simulink model "DC_DC_source_based_matrix_switches1"  (R2023b)
settings: Solver=FixedStepAuto  StartTime=0.0  StopTime=10000  FixedStep=0.01  RelTol=1e-3
InitFcn:
  | %run('D:\Thesis\main.m')
  | %run('E:\Thesis\main.m')
values from neighbouring files (symbols this model uses):
  cell_cap_Ah = 2.2    [find_maximum_ovlp.m]    (also in main.m)
  dst_q_cls = zeros(50, 2)    [main.m]
  dst_trg_soc_av = zeros(50, 1)    [main.m]
  soc = soc_in    [balance_costF.m]    (also in find_maximum_ovlp.m = fix(rand (1, cell_count) * 100); log_clustering.m; main.m = [16   16  50  27  27  23  22  73  73]; plot_final.m)
  src_q_cls = zeros(50, 2)    [main.m]
  src_trg_soc_av = zeros(50, 1)    [main.m]
undefined symbols (not defined in the file or in its folder): Ion, Lithium
libraries: spsIdealSwitchLib x18, spsBatteryLib x10, spsControlledCurrentSourceLib x4, spsVoltageMeasurementLib x4, simulink x2, slpidlib x1, spspowerguiLib x1
(part 1 of 2)
settings Model: NumberOfSteps=500  Creator=Mahdi  LastModifiedBy=Mahdi
settings OptimizationCC: DefaultParameterBehavior=Inlined  EnhancedBackFolding=on  PassReuseOutputArgsAs=Individual arguments  ZeroExternalMemoryAtStartup=off  ZeroInternalMemoryAtStartup=off  OptimizeBlockOrder=speed  DifferentSizesBufferReuse=on  OptimizationCustomize=off  EfficientTunableParamExpr=on
settings DebuggingCC: ParameterTunabilityLossMsg=error
settings HardwareCC: ProdBitPerInt=16  ProdBitPerPointer=16  ProdBitPerSizeT=16  ProdBitPerPtrDiffT=16  ProdLargestAtomicFloat=None  ProdWordSize=16  ProdHWDeviceType=STMicroelectronics->ST10/Super10
settings ModelReferenceCC: ModelReferenceMinAlgLoopOccurrences=on
settings SFSimCC: MATLABDynamicMemAlloc=off
settings RTWCC: Description=Embedded Coder  SystemTargetFile=ert.tlc  TemplateMakefile=ert_default_tmf
settings CodeAppCC: ForceParamTrailComments=on  IgnoreCustomStorageClasses=off  OperatorAnnotations=on  SimulinkDataObjDesc=on  SFDataObjDesc=on  InsertBlockDesc=on
settings ERTTargetCC: TargetLangStandard=C99 (ISO)  GenerateSampleERTMain=on  SupportContinuousTime=on  SupportVariableSizeSignals=on  InlinedParameterPlacement=NonHierarchical  ERTCustomFileTemplate=example_file_process.tlc

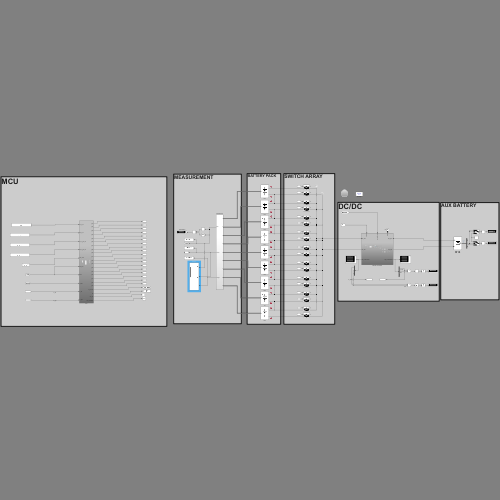
[thumbnail: Simulink's stored preview of the top-level diagram]
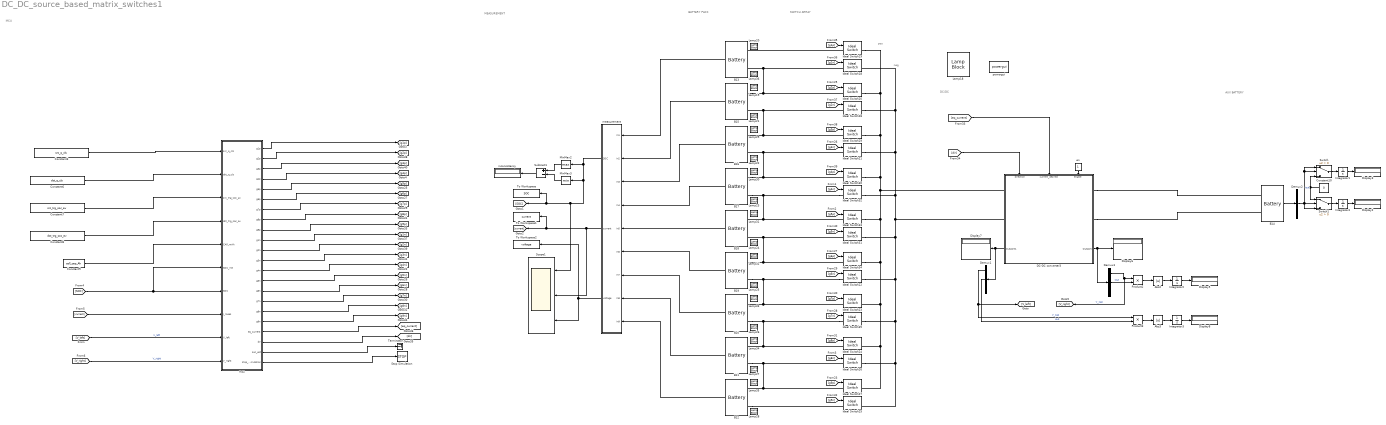
== system DC_DC_source_based_matrix_switches1 ==
  note: MEASUREMENT
  note: DC/DC
  note: SWITCH ARRAY
  note: pos
  note: BATTERY PACK
  note: neg
  note: AUX BATTERY
  note: MCU
  Abs2 : Abs  SaturateOnIntegerOverflow=off
  Abs3 : Abs  SaturateOnIntegerOverflow=off
  B11 : spsBatteryLib/Battery  BatType=Lithium-Ion  ShowTempParam=off  ThermalPreset=no  ShowAgeParam=off  NomV=3.7  NomQ=2.2  SOC=soc(1, 8)  Batt_Tr=30  PresetModel=on  MaxQ=2.2  MinV=2.775  FullV=4.3068  Dis_rate=0.95652  R=0.016818  Normal_OP=1.9896  expZone="[3.9974     0.10809]"  current=[6.5 13 32.5]  Units=Time  Tci=20  NomT=20  T2=-30  MaxQ2=4.8  FullV2=7.1  Normal_OP2=5.655  expZone2="[6.58           1]"  Rca=0.6  ti=2000  Dp=0  Neq0=0  Tsim=1e6  Ta1=25  Qeol=5.4*0.9  Reol=0.013333*1.2  Char_age=[2.3478, 3]  Dis_age=[2.3478, 10]  N1=1500  N2=10500  N3=1000  N4=1400  Ta2=45  N5=950
  B12 : spsBatteryLib/Battery  BatType=Lithium-Ion  ShowTempParam=off  ThermalPreset=no  ShowAgeParam=off  NomV=3.7  NomQ=2.2  SOC=soc(1, 9)  Batt_Tr=30  PresetModel=on  MaxQ=2.2  MinV=2.775  FullV=4.3068  Dis_rate=0.95652  R=0.016818  Normal_OP=1.9896  expZone="[3.9974     0.10809]"  current=[6.5 13 32.5]  Units=Time  Tci=20  NomT=20  T2=-30  MaxQ2=4.8  FullV2=7.1  Normal_OP2=5.655  expZone2="[6.58           1]"  Rca=0.6  ti=2000  Dp=0  Neq0=0  Tsim=1e6  Ta1=25  Qeol=5.4*0.9  Reol=0.013333*1.2  Char_age=[2.3478, 3]  Dis_age=[2.3478, 10]  N1=1500  N2=10500  N3=1000  N4=1400  Ta2=45  N5=950
  B13 : spsBatteryLib/Battery  BatType=Lithium-Ion  ShowTempParam=off  ThermalPreset=no  ShowAgeParam=off  NomV=3.7  NomQ=2.2  SOC=soc(1, 1)  Batt_Tr=30  PresetModel=on  MaxQ=2.2  MinV=2.775  FullV=4.3068  Dis_rate=0.95652  R=0.016818  Normal_OP=1.9896  expZone="[3.9974     0.10809]"  current=[6.5 13 32.5]  Units=Time  Tci=20  NomT=20  T2=-30  MaxQ2=4.8  FullV2=7.1  Normal_OP2=5.655  expZone2="[6.58           1]"  Rca=0.6  ti=2000  Dp=0  Neq0=0  Tsim=1e6  Ta1=25  Qeol=5.4*0.9  Reol=0.013333*1.2  Char_age=[2.3478, 3]  Dis_age=[2.3478, 10]  N1=1500  N2=10500  N3=1000  N4=1400  Ta2=45  N5=950
  B14 : spsBatteryLib/Battery  BatType=Lithium-Ion  ShowTempParam=off  ThermalPreset=no  ShowAgeParam=off  NomV=12  NomQ=60  SOC=soc(1, 1)  Batt_Tr=30  PresetModel=on  MaxQ=60  MinV=9  FullV=13.9678  Dis_rate=26.087  R=0.002  Normal_OP=54.2609  expZone="[12.9646      2.94783]"  current=[6.5 13 32.5]  Units=Time  Tci=20  NomT=20  T2=-30  MaxQ2=4.8  FullV2=7.1  Normal_OP2=5.655  expZone2="[6.58           1]"  Rca=0.6  ti=2000  Dp=0  Neq0=0  Tsim=1e6  Ta1=25  Qeol=5.4*0.9  Reol=0.013333*1.2  Char_age=[2.3478, 3]  Dis_age=[2.3478, 10]  N1=1500  N2=10500  N3=1000  N4=1400  Ta2=45  N5=950
  B15 : spsBatteryLib/Battery  BatType=Lithium-Ion  ShowTempParam=off  ThermalPreset=no  ShowAgeParam=off  NomV=3.7  NomQ=2.2  SOC=soc(1, 2)  Batt_Tr=30  PresetModel=on  MaxQ=2.2  MinV=2.775  FullV=4.3068  Dis_rate=0.95652  R=0.016818  Normal_OP=1.9896  expZone="[3.9974     0.10809]"  current=[6.5 13 32.5]  Units=Time  Tci=20  NomT=20  T2=-30  MaxQ2=4.8  FullV2=7.1  Normal_OP2=5.655  expZone2="[6.58           1]"  Rca=0.6  ti=2000  Dp=0  Neq0=0  Tsim=1e6  Ta1=25  Qeol=5.4*0.9  Reol=0.013333*1.2  Char_age=[2.3478, 3]  Dis_age=[2.3478, 10]  N1=1500  N2=10500  N3=1000  N4=1400  Ta2=45  N5=950
  B16 : spsBatteryLib/Battery  BatType=Lithium-Ion  ShowTempParam=off  ThermalPreset=no  ShowAgeParam=off  NomV=3.7  NomQ=2.2  SOC=soc(1, 3)  Batt_Tr=30  PresetModel=on  MaxQ=2.2  MinV=2.775  FullV=4.3068  Dis_rate=0.95652  R=0.016818  Normal_OP=1.9896  expZone="[3.9974     0.10809]"  current=[6.5 13 32.5]  Units=Time  Tci=20  NomT=20  T2=-30  MaxQ2=4.8  FullV2=7.1  Normal_OP2=5.655  expZone2="[6.58           1]"  Rca=0.6  ti=2000  Dp=0  Neq0=0  Tsim=1e6  Ta1=25  Qeol=5.4*0.9  Reol=0.013333*1.2  Char_age=[2.3478, 3]  Dis_age=[2.3478, 10]  N1=1500  N2=10500  N3=1000  N4=1400  Ta2=45  N5=950
  B17 : spsBatteryLib/Battery  BatType=Lithium-Ion  ShowTempParam=off  ThermalPreset=no  ShowAgeParam=off  NomV=3.7  NomQ=2.2  SOC=soc(1, 4)  Batt_Tr=30  PresetModel=on  MaxQ=2.2  MinV=2.775  FullV=4.3068  Dis_rate=0.95652  R=0.016818  Normal_OP=1.9896  expZone="[3.9974     0.10809]"  current=[6.5 13 32.5]  Units=Time  Tci=20  NomT=20  T2=-30  MaxQ2=4.8  FullV2=7.1  Normal_OP2=5.655  expZone2="[6.58           1]"  Rca=0.6  ti=2000  Dp=0  Neq0=0  Tsim=1e6  Ta1=25  Qeol=5.4*0.9  Reol=0.013333*1.2  Char_age=[2.3478, 3]  Dis_age=[2.3478, 10]  N1=1500  N2=10500  N3=1000  N4=1400  Ta2=45  N5=950
  B18 : spsBatteryLib/Battery  BatType=Lithium-Ion  ShowTempParam=off  ThermalPreset=no  ShowAgeParam=off  NomV=3.7  NomQ=2.2  SOC=soc(1, 5)  Batt_Tr=30  PresetModel=on  MaxQ=2.2  MinV=2.775  FullV=4.3068  Dis_rate=0.95652  R=0.016818  Normal_OP=1.9896  expZone="[3.9974     0.10809]"  current=[6.5 13 32.5]  Units=Time  Tci=20  NomT=20  T2=-30  MaxQ2=4.8  FullV2=7.1  Normal_OP2=5.655  expZone2="[6.58           1]"  Rca=0.6  ti=2000  Dp=0  Neq0=0  Tsim=1e6  Ta1=25  Qeol=5.4*0.9  Reol=0.013333*1.2  Char_age=[2.3478, 3]  Dis_age=[2.3478, 10]  N1=1500  N2=10500  N3=1000  N4=1400  Ta2=45  N5=950
  B19 : spsBatteryLib/Battery  BatType=Lithium-Ion  ShowTempParam=off  ThermalPreset=no  ShowAgeParam=off  NomV=3.7  NomQ=2.2  SOC=soc(1, 6)  Batt_Tr=30  PresetModel=on  MaxQ=2.2  MinV=2.775  FullV=4.3068  Dis_rate=0.95652  R=0.016818  Normal_OP=1.9896  expZone="[3.9974     0.10809]"  current=[6.5 13 32.5]  Units=Time  Tci=20  NomT=20  T2=-30  MaxQ2=4.8  FullV2=7.1  Normal_OP2=5.655  expZone2="[6.58           1]"  Rca=0.6  ti=2000  Dp=0  Neq0=0  Tsim=1e6  Ta1=25  Qeol=5.4*0.9  Reol=0.013333*1.2  Char_age=[2.3478, 3]  Dis_age=[2.3478, 10]  N1=1500  N2=10500  N3=1000  N4=1400  Ta2=45  N5=950
  B20 : spsBatteryLib/Battery  BatType=Lithium-Ion  ShowTempParam=off  ThermalPreset=no  ShowAgeParam=off  NomV=3.7  NomQ=2.2  SOC=soc(1, 7)  Batt_Tr=30  PresetModel=on  MaxQ=2.2  MinV=2.775  FullV=4.3068  Dis_rate=0.95652  R=0.016818  Normal_OP=1.9896  expZone="[3.9974     0.10809]"  current=[6.5 13 32.5]  Units=Time  Tci=20  NomT=20  T2=-30  MaxQ2=4.8  FullV2=7.1  Normal_OP2=5.655  expZone2="[6.58           1]"  Rca=0.6  ti=2000  Dp=0  Neq0=0  Tsim=1e6  Ta1=25  Qeol=5.4*0.9  Reol=0.013333*1.2  Char_age=[2.3478, 3]  Dis_age=[2.3478, 10]  N1=1500  N2=10500  N3=1000  N4=1400  Ta2=45  N5=950
  Constant10 : Constant  Value=0
  Constant3 : Constant  Value=src_q_cls
  Constant6 : Constant  Value=dst_q_cls
  Constant7 : Constant  Value=src_trg_soc_av
  Constant8 : Constant  Value=dst_trg_soc_av
  Constant9 : Constant  Value=cell_cap_Ah
  DC-DC converter3 : Subsystem
      settings: PortSchema="{\"entries\":[{\"content\":{\"sides\":[{\"content\":{\"connectorIds\":[\"LConn1\",\"LConn2\",\"Out2\"]},\"type\":\"ConnectorPlacement.EquallySpacedRectSide\",\"uuid\":\"b8e9ea21-fc6f-4abe-9815-7c96c8754cc1\"},{\"content\":{\"connectorIds\":[\"RConn1\",\"RConn2\",\"Out1\"],\"side\":\"RIGHT\"},\"type\":\"ConnectorPlacement.EquallySpacedRectSide\",\"uuid\":\"546bb611-6f28-45af-a15a-a960a3093258\"},{\"content\":{\"connectorIds\":[\"In1\",\"In2\",\"In3\"],\"side\":\"TOP\"},\"type\":\"ConnectorPlacement.EquallySpacedRectSide\",\"uuid\":\"f1a81754-76ae-41da-bcef-17d54c1fc977\"}]},\"type\":\"ConnectorPlacement.EquallySpacedConnector\",\"uuid\":\"f395fac5-4dd1-431a-bb8e-7682cfb9cc98\"}],\"packageUris\":[\"http://schema.mathworks.com/mf0/Connector/R2020b\"],\"version\":\"1.0\"}"
  Demux1 : Demux  Outputs=3
  Demux2 : Demux  Outputs=3
  Demux3 : Demux  Outputs=3
  Display{2..3,5..8} (6 alike) : Display
  Ideal Switch{18..35} (18 alike) : spsIdealSwitchLib/Ideal Switch  Ron=0.001  Lon=0  IC=0  Rs=1e5  Cs=inf  Measurements=on
  Integrator{1..4} (4 alike) : Integrator
  Lamp{18..36} (19 alike) : LampBlock  LabelPosition=Hide
  MinMax2 : MinMax  Function=max
  MinMax3 : MinMax
  Product2 : Product
  Product3 : Product
  Scope1 : Scope  NumInputPorts=3
  Stop Simulation : Stop
  Subtract1 : Sum  Inputs=+-
  Switch : Switch  Criteria=u2 > Threshold  SaturateOnIntegerOverflow=off  InputSameDT=off
  Switch1 : Switch  Criteria=u2 > Threshold  SaturateOnIntegerOverflow=off  InputSameDT=off
  Terminator : Terminator
  To Workspace : ToWorkspace  VariableName=SOC  SaveFormat=Timeseries  SampleTime=-1
      settings: Decimation=10
  To Workspace1 : ToWorkspace  VariableName=current  SaveFormat=Timeseries  SampleTime=-1
      settings: Decimation=10
  To Workspace2 : ToWorkspace  VariableName=voltage  SaveFormat=Timeseries  SampleTime=-1
      settings: Decimation=10
  en : Constant
  inconsistency : Display
  mcu : Subsystem
  measurement : Subsystem
  powergui : spspowerguiLib/powergui  Priority=1  SimulationMode=Discrete  SampleTime=1E-1  frequency=60  Iterations=50  frequencyindice=0  Pbase=100e6  ErrMax=1e-4  UnitsV=kV  UnitsW=MW  buscounter=0  FunctionMessages=off  echomessages=off  EnableUseOfTLC=off  CurrentSourceSwitches=off  DisableSnubberDevices=off  DisableRonSwitches=off  DisableVfSwitches=off  DisplayEquations=off  AutomaticDiscreteSolvers=off  SolverType=Tustin/Backward Euler (TBE)  Interpol=off  ExternalGateDelay=off  methode=on  Ts=1000  x0status=blocks  SPID=off  SwTol=0  HookPort=off  NonlinearTolerance=1e-4  nMaxIteration=10  ContinueOnMaxIteration=off  RestoreLinks=warning  ResistiveCurrentMeasurement=off  Frange=[0:2:500]  Ylog=off  Xlog=on  ShowGrid=off  save=off  variable=ZData  structure=0  ZoomFFT=off  StartTime=0.0  cycles=1  DisplayStyle=1  fundamental=60  FreqAxis=off  MaxFrequency=1000  frequencyindicesteady=1  RmsSteady=1  display=off
  wires:
  [g8n] -> Ideal Switch26/1
  Demux3/2 -> Product2/2  "Iout"
  measurement/1(SOC) -> MinMax2/1, MinMax3/1, Scope1/1, To Workspace/1, [SOC]
  [g2n] -> Ideal Switch28/1
  B11/1 -> measurement/8(In8)
  [g6n] -> Ideal Switch22/1
  MinMax3/1 -> Subtract1/2
  Demux1/2 -> Product3/2  "Iout"
  Product3/1 -> Abs3/1
  Subtract1/1 -> inconsistency/1
  [g9p] -> Ideal Switch27/1
  [g6p] -> Ideal Switch34/1
  B12/1 -> measurement/9(In9)
  [g5n] -> Ideal Switch31/1
  B20/1 -> measurement/7(In7)
  Demux1/1 -> [V_left], Product3/1  "V_cap"
  B19/1 -> measurement/6(In6)
  [g2p] -> Ideal Switch20/1
  [g8p] -> Ideal Switch24/1
  Abs2/1 -> Integrator2/1
  B15/1 -> measurement/2(In2)
  [g7n] -> Ideal Switch35/1
  [g4n] -> Ideal Switch32/1
  [g4p] -> Ideal Switch30/1
  measurement/2(current) -> Scope1/2, To Workspace1/1, [current]
  B18/1 -> measurement/5(In5)
  Product2/1 -> Abs2/1
  DC-DC converter3/1(Outport) -> Display6/1, Demux3/1
  MinMax2/1 -> Subtract1/1
  Integrator2/1 -> Display5/1
  [g1n] -> Ideal Switch18/1
  Integrator3/1 -> Display8/1
  Abs3/1 -> Integrator3/1
  [g5p] -> Ideal Switch33/1
  [g9n] -> Ideal Switch25/1
  B16/1 -> measurement/3(In3)
  [g1p] -> Ideal Switch19/1
  B17/1 -> measurement/4(In4)
  B13/1 -> measurement/1(In1)
  DC-DC converter3/2(Outport1) -> Display7/1, Demux1/1
  Demux3/1 -> [V_right], Product2/1  "V_cap"
  [g3p] -> Ideal Switch29/1
  [g3n] -> Ideal Switch21/1
  [g7p] -> Ideal Switch23/1
  measurement/3(voltage) -> To Workspace2/1, Scope1/3
  Integrator1/1 -> Display3/1
  Switch/1 -> Integrator1/1
  Integrator4/1 -> Display2/1
  B14/1 -> Demux2/1
  Demux2/2 -> Switch1/3, Switch1/2, Switch/1, Switch/2  "Iout"
  Switch1/1 -> Integrator4/1
  Constant10/1 -> Switch1/1, Switch/3
  [dir] -> DC-DC converter3/1(direction)
  en/1 -> DC-DC converter3/3(enable)
  Constant9/1 -> mcu/5(CAP_mAh)
  Constant7/1 -> mcu/3(src_trg_soc_av)
  Constant3/1 -> mcu/1(src_q_cls)
  Constant6/1 -> mcu/2(dst_q_cls)
  Constant8/1 -> mcu/4(dst_trg_soc_av)
  [SOC] -> mcu/6(SOC_init), mcu/7(SOC)
  [current] -> mcu/8(I_meas)
  mcu/13(g4n) -> [g4n]
  mcu/18(g9n) -> [g9n]
  mcu/19(eq_current) -> [eq_current]
  mcu/20(dir) -> [dir]
  mcu/17(g8n) -> [g8n]
  mcu/16(g7n) -> [g7n]
  mcu/15(g6n) -> [g6n]
  mcu/12(g3n) -> [g3n]
  mcu/14(g5n) -> [g5n]
  mcu/10(g1n) -> [g1n]
  mcu/11(g2n) -> [g2n]
  mcu/9(g9p) -> [g9p]
  mcu/8(g8p) -> [g8p]
  mcu/7(g7p) -> [g7p]
  mcu/6(g6p) -> [g6p]
  mcu/5(g5p) -> [g5p]
  mcu/4(g4p) -> [g4p]
  mcu/3(g3p) -> [g3p]
  mcu/2(g2p) -> [g2p]
  mcu/1(g1p) -> [g1p]
  mcu/21(soc_est) -> Terminator/1
  mcu/22(stop_simulation) -> Stop Simulation/1
  [eq_current] -> DC-DC converter3/2(current_desired)
  [V_left] -> mcu/9(V_left)  "V_left"
  [V_right] -> mcu/10(V_right)  "V_right"
  connections:
  B18/LConn2 -- Ideal Switch34/LConn1 -- B19/LConn1 -- Ideal Switch31/LConn1
  Ideal Switch29/RConn1 -- DC-DC converter3/LConn1 -- Ideal Switch23/RConn1 -- Ideal Switch27/RConn1 -- Ideal Switch24/RConn1 -- Ideal Switch34/RConn1 -- Ideal Switch33/RConn1 -- Ideal Switch30/RConn1 -- Ideal Switch19/RConn1 -- Ideal Switch20/RConn1
  Ideal Switch32/RConn1 -- Ideal Switch18/RConn1 -- Ideal Switch28/RConn1 -- Ideal Switch21/RConn1 -- DC-DC converter3/LConn2 -- Ideal Switch22/RConn1 -- Ideal Switch26/RConn1 -- Ideal Switch25/RConn1 -- Ideal Switch35/RConn1 -- Ideal Switch31/RConn1
  B15/LConn1 -- B13/LConn2 -- Ideal Switch18/LConn1 -- Ideal Switch20/LConn1
  Ideal Switch35/LConn1 -- Ideal Switch24/LConn1 -- B11/LConn1 -- B20/LConn2
  Ideal Switch21/LConn1 -- B16/LConn2 -- B17/LConn1 -- Ideal Switch30/LConn1
  Ideal Switch22/LConn1 -- B20/LConn1 -- Ideal Switch23/LConn1 -- B19/LConn2
  Ideal Switch32/LConn1 -- B18/LConn1 -- Ideal Switch33/LConn1 -- B17/LConn2
  Ideal Switch29/LConn1 -- B16/LConn1 -- Ideal Switch28/LConn1 -- B15/LConn2
  B12/LConn1 -- Ideal Switch27/LConn1 -- Ideal Switch26/LConn1 -- B11/LConn2
  Ideal Switch19/LConn1 -- B13/LConn1
  DC-DC converter3/RConn1 -- B14/LConn1
  B12/LConn2 -- Ideal Switch25/LConn1
  DC-DC converter3/RConn2 -- B14/LConn2

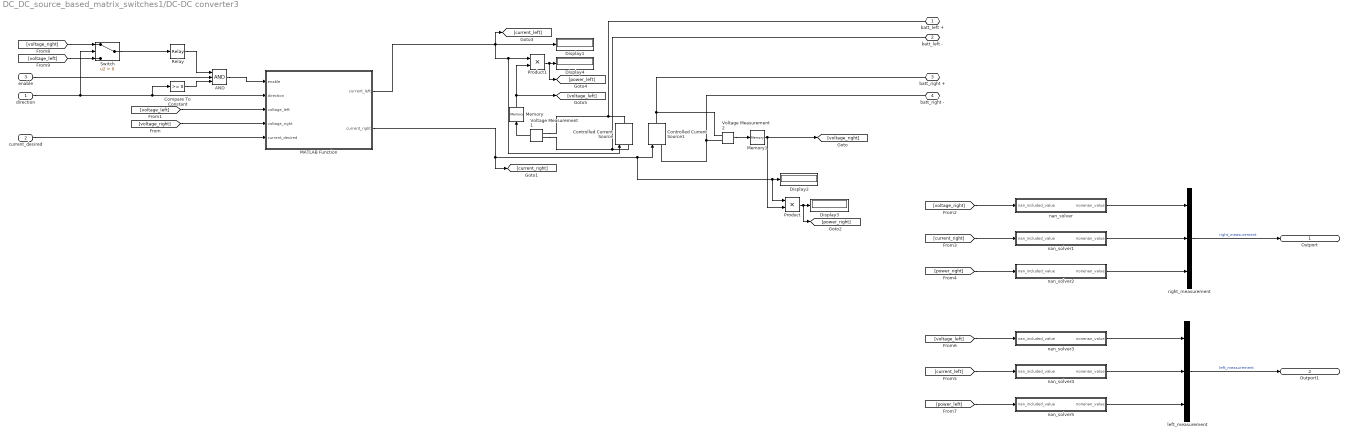
== system DC_DC_source_based_matrix_switches1/DC-DC converter3 ==
  direction : Inport
  current_desired : Inport  Port=2
  enable : Inport  Port=3
  AND : Logic  Inputs=3  IconShape=distinctive  AllPortsSameDT=off  OutDataTypeStr=boolean
  Compare To Constant : simulink/Logic and Bit Operations/Compare To Constant  relop=>=  const=0  OutDataTypeStr=boolean
  Controlled Current Source : spsControlledCurrentSourceLib/Controlled Current Source  Initialize=on  Source_Type=DC  Amplitude=0  Phase=0  Frequency=0  Measurements=None
  Controlled Current Source1 : spsControlledCurrentSourceLib/Controlled Current Source  Initialize=on  Source_Type=AC  Amplitude=0  Phase=0  Frequency=0  Measurements=None
  Display{1..4} (4 alike) : Display
  MATLAB Function : MATLAB Function  TreatAsAtomicUnit=on
  Memory : Memory
  Memory1 : Memory
  Product : Product
  Product1 : Product
  Relay : Relay  OnSwitchValue=3.5  OffSwitchValue=2
  Switch : Switch  Criteria=u2 > Threshold  SaturateOnIntegerOverflow=off  InputSameDT=off
  Voltage Measurement1 : spsVoltageMeasurementLib/Voltage Measurement  PhasorSimulation=off  OutputType=Complex  PSBequivalent=0
  Voltage Measurement2 : spsVoltageMeasurementLib/Voltage Measurement  PhasorSimulation=off  OutputType=Complex  PSBequivalent=0
  left_measurement : Mux  Inputs=3
  nan_solver : Subsystem
  nan_solver1 : Subsystem
  nan_solver2 : Subsystem
  nan_solver3 : Subsystem
  nan_solver4 : Subsystem
  nan_solver5 : Subsystem
  right_measurement : Mux  Inputs=3
  batt_left + : PMIOPort  Side=Left
  batt_left - : PMIOPort  Port=2  Side=Left
  batt_right + : PMIOPort  Port=3  Side=Right
  batt_right - : PMIOPort  Port=4  Side=Right
  Outport : Outport
  Outport1 : Outport  Port=2
  wires:
  MATLAB Function/1(current_left) -> Controlled Current Source/1, Product1/1, [current_left], Display1/1
  enable/1 -> AND/2
  Voltage Measurement2/1 -> Memory1/1
  direction/1 -> Compare To Constant/1, MATLAB Function/2(direction), Switch/2
  [voltage_right] -> MATLAB Function/4(voltage_right)
  [voltage_left] -> MATLAB Function/3(voltage_left)
  Product/1 -> [power_right], Display3/1
  Product1/1 -> [power_left], Display4/1
  [voltage_right] -> nan_solver/1(nan_included_value)
  [current_right] -> nan_solver1/1(nan_included_value)
  [power_right] -> nan_solver2/1(nan_included_value)
  [power_left] -> nan_solver5/1(nan_included_value)
  [current_left] -> nan_solver4/1(nan_included_value)
  [voltage_left] -> nan_solver3/1(nan_included_value)
  right_measurement/1 -> Outport/1  "right_measurement"
  left_measurement/1 -> Outport1/1  "left_measurement"
  Voltage Measurement1/1 -> Memory/1
  Relay/1 -> AND/1
  AND/1 -> MATLAB Function/1(enable)
  Switch/1 -> Relay/1
  [voltage_left] -> Switch/3
  [voltage_right] -> Switch/1
  Memory/1 -> Product1/2, [voltage_left]
  Memory1/1 -> [voltage_right], Product/2
  Compare To Constant/1 -> AND/3
  MATLAB Function/2(current_right) -> [current_right], Product/1, Display2/1, Controlled Current Source1/1
  current_desired/1 -> MATLAB Function/5(current_desired)
  nan_solver/1(nonenan_value) -> right_measurement/1
  nan_solver1/1(nonenan_value) -> right_measurement/2
  nan_solver2/1(nonenan_value) -> right_measurement/3
  nan_solver3/1(nonenan_value) -> left_measurement/1
  nan_solver4/1(nonenan_value) -> left_measurement/2
  nan_solver5/1(nonenan_value) -> left_measurement/3
  connections:
  Voltage Measurement1/LConn1 -- batt_left +/RConn1 -- Controlled Current Source/RConn1
  Controlled Current Source1/RConn1 -- batt_right +/RConn1 -- Voltage Measurement2/LConn1
  Voltage Measurement2/LConn2 -- Controlled Current Source1/LConn1 -- batt_right -/RConn1
  Voltage Measurement1/LConn2 -- batt_left -/RConn1 -- Controlled Current Source/LConn1

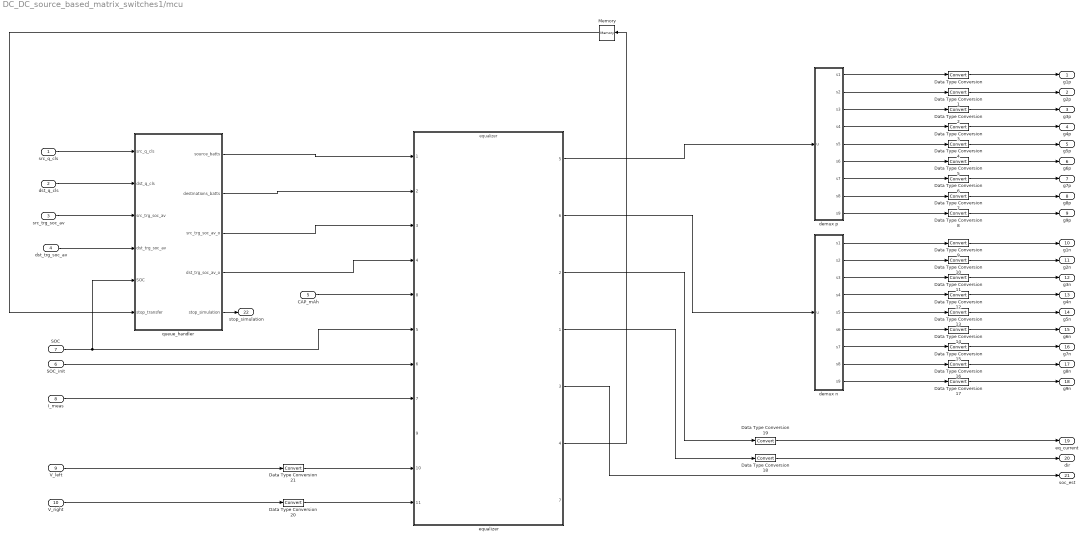
== system DC_DC_source_based_matrix_switches1/mcu ==
  src_q_cls : Inport
  dst_q_cls : Inport  Port=2
  src_trg_soc_av : Inport  Port=3
  dst_trg_soc_av : Inport  Port=4
  CAP_mAh : Inport  Port=5  PortDimensions=[1 1]
  SOC_init : Inport  Port=6
  SOC : Inport  Port=7
  I_meas : Inport  Port=8
  V_left : Inport  Port=9
  V_right : Inport  Port=10
  Data Type Conversion{,1..21} (22 alike) : DataTypeConversion  SaturateOnIntegerOverflow=off  RndMeth=Floor
  Memory : Memory
  demux n : MATLAB Function  TreatAsAtomicUnit=on
  demux p : MATLAB Function  TreatAsAtomicUnit=on
  equalizer : ModelReference  ModelNameDialog=equalizer.slx  SimulationMode=Normal  ModelReferenceVersion=4.57
      settings: PortSchema="{\"entries\":[{\"content\":{\"sides\":[{\"content\":{\"connectorIds\":[\"In1\",\"In2\",\"In3\",\"In4\",\"In8\",\"In5\",\"In6\",\"In7\",\"In9\",\"In10\",\"In11\"]},\"type\":\"ConnectorPlacement.EquallySpacedRectSide\",\"uuid\":\"0e6c575f-ddf8-42c7-9de1-4e19b4f5acff\"},{\"content\":{\"connectorIds\":[\"Out5\",\"Out6\",\"Out2\",\"Out1\",\"Out3\",\"Out4\",\"Out7\"],\"side\":\"RIGHT\"},\"type\":\"ConnectorPlacement.EquallySpacedRectSide\",\"uuid\":\"ffa8e601-c4c1-438b-9d74-db810c4522c7\"},{\"content\":{\"side\":\"TOP\"},\"type\":\"ConnectorPlacement.EquallySpacedRectSide\",\"uuid\":\"66088ef6-14ba-4cc7-bf73-23eeb83a4754\"}]},\"type\":\"ConnectorPlacement.EquallySpacedConnector\",\"uuid\":\"d6774570-3838-464e-8129-9c381a0fca30\"}],\"packageUris\":[\"http://schema.mathworks.com/mf0/Connector/R2020b\"],\"version\":\"1.0\"}"
  queue_handler : MATLAB Function  TreatAsAtomicUnit=on
  g1p : Outport  PortDimensions=1
  g2p : Outport  Port=2
  g3p : Outport  Port=3
  g4p : Outport  Port=4
  g5p : Outport  Port=5
  g6p : Outport  Port=6
  g7p : Outport  Port=7
  g8p : Outport  Port=8
  g9p : Outport  Port=9
  g1n : Outport  Port=10
  g2n : Outport  Port=11
  g3n : Outport  Port=12
  g4n : Outport  Port=13
  g5n : Outport  Port=14
  g6n : Outport  Port=15
  g7n : Outport  Port=16
  g8n : Outport  Port=17
  g9n : Outport  Port=18
  eq_current : Outport  Port=19
  dir : Outport  Port=20
  soc_est : Outport  Port=21  PortDimensions=[1 9]
  stop_simulation : Outport  Port=22  PortDimensions=1
  wires:
  equalizer/2 -> Data Type Conversion19/1
  equalizer/1 -> Data Type Conversion18/1
  equalizer/3 -> soc_est/1
  equalizer/4 -> Memory/1
  SOC/1 -> equalizer/5, queue_handler/5(SOC)
  SOC_init/1 -> equalizer/6
  I_meas/1 -> equalizer/7
  CAP_mAh/1 -> equalizer/8
  src_q_cls/1 -> queue_handler/1(src_q_cls)
  dst_q_cls/1 -> queue_handler/2(dst_q_cls)
  src_trg_soc_av/1 -> queue_handler/3(src_trg_soc_av)
  dst_trg_soc_av/1 -> queue_handler/4(dst_trg_soc_av)
  queue_handler/1(source_batts) -> equalizer/1
  queue_handler/2(destinations_batts) -> equalizer/2
  queue_handler/3(src_trg_soc_av_o) -> equalizer/3
  queue_handler/4(dst_trg_soc_av_o) -> equalizer/4
  Memory/1 -> queue_handler/6(stop_transfer)
  Data Type Conversion18/1 -> dir/1
  Data Type Conversion19/1 -> eq_current/1
  queue_handler/5(stop_simulation) -> stop_simulation/1
  Data Type Conversion/1 -> g1p/1
  Data Type Conversion1/1 -> g2p/1
  Data Type Conversion2/1 -> g3p/1
  Data Type Conversion3/1 -> g4p/1
  Data Type Conversion4/1 -> g5p/1
  Data Type Conversion5/1 -> g6p/1
  Data Type Conversion6/1 -> g7p/1
  Data Type Conversion7/1 -> g8p/1
  Data Type Conversion8/1 -> g9p/1
  Data Type Conversion9/1 -> g1n/1
  Data Type Conversion10/1 -> g2n/1
  Data Type Conversion11/1 -> g3n/1
  Data Type Conversion12/1 -> g4n/1
  Data Type Conversion13/1 -> g5n/1
  Data Type Conversion14/1 -> g6n/1
  Data Type Conversion15/1 -> g7n/1
  Data Type Conversion16/1 -> g8n/1
  Data Type Conversion17/1 -> g9n/1
  demux p/5(s5) -> Data Type Conversion4/1
  demux p/8(s8) -> Data Type Conversion7/1
  demux p/9(s9) -> Data Type Conversion8/1
  demux p/7(s7) -> Data Type Conversion6/1
  equalizer/6 -> demux n/1(u)
  demux p/4(s4) -> Data Type Conversion3/1
  demux p/1(s1) -> Data Type Conversion/1
  demux p/6(s6) -> Data Type Conversion5/1
  demux p/2(s2) -> Data Type Conversion1/1
  demux n/3(s3) -> Data Type Conversion11/1
  demux n/5(s5) -> Data Type Conversion13/1
  demux p/3(s3) -> Data Type Conversion2/1
  demux n/9(s9) -> Data Type Conversion17/1
  demux n/6(s6) -> Data Type Conversion14/1
  demux n/4(s4) -> Data Type Conversion12/1
  demux n/7(s7) -> Data Type Conversion15/1
  demux n/1(s1) -> Data Type Conversion9/1
  demux n/8(s8) -> Data Type Conversion16/1
  demux n/2(s2) -> Data Type Conversion10/1
  equalizer/5 -> demux p/1(u)
  V_left/1 -> Data Type Conversion21/1
  V_right/1 -> Data Type Conversion20/1
  Data Type Conversion21/1 -> equalizer/10
  Data Type Conversion20/1 -> equalizer/11

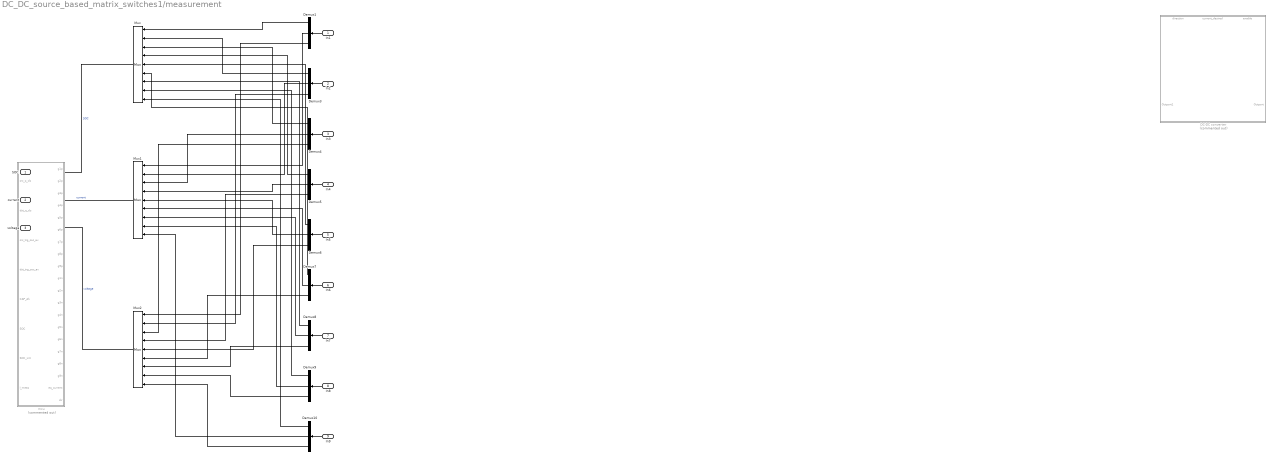
== system DC_DC_source_based_matrix_switches1/measurement ==
  In1 : Inport
  In2 : Inport  Port=2
  In3 : Inport  Port=3
  In4 : Inport  Port=4
  In5 : Inport  Port=5
  In6 : Inport  Port=6
  In7 : Inport  Port=7
  In8 : Inport  Port=8
  In9 : Inport  Port=9
  DC-DC converter : Subsystem  Commented=on
      settings: PortSchema="{\"entries\":[{\"content\":{\"sides\":[{\"content\":{\"connectorIds\":[\"LConn1\",\"LConn2\",\"Out2\"]},\"type\":\"ConnectorPlacement.EquallySpacedRectSide\",\"uuid\":\"b8e9ea21-fc6f-4abe-9815-7c96c8754cc1\"},{\"content\":{\"connectorIds\":[\"RConn1\",\"RConn2\",\"Out1\"],\"side\":\"RIGHT\"},\"type\":\"ConnectorPlacement.EquallySpacedRectSide\",\"uuid\":\"546bb611-6f28-45af-a15a-a960a3093258\"},{\"content\":{\"connectorIds\":[\"In1\",\"In2\",\"In3\"],\"side\":\"TOP\"},\"type\":\"ConnectorPlacement.EquallySpacedRectSide\",\"uuid\":\"f1a81754-76ae-41da-bcef-17d54c1fc977\"}]},\"type\":\"ConnectorPlacement.EquallySpacedConnector\",\"uuid\":\"f395fac5-4dd1-431a-bb8e-7682cfb9cc98\"}],\"packageUris\":[\"http://schema.mathworks.com/mf0/Connector/R2020b\"],\"version\":\"1.0\"}"
  Demux{1,3..10} (9 alike) : Demux  Outputs=3
  Mux : Mux  Inputs=9
  Mux1 : Mux  Inputs=9
  Mux2 : Mux  Inputs=9
  mcu : Subsystem  Commented=on
  SOC : Outport
  current : Outport  Port=2
  voltage : Outport  Port=3
  wires:
  In7/1 -> Demux8/1
  Demux6/3 -> Mux2/5
  Demux8/3 -> Mux2/7
  In5/1 -> Demux6/1
  Demux7/3 -> Mux2/6
  Demux4/1 -> Mux/3
  Demux10/3 -> Mux2/9
  Mux1/1 -> current/1  "current"
  Demux4/2 -> Mux1/3
  Demux1/3 -> Mux2/1
  Demux5/3 -> Mux2/4
  Demux10/1 -> Mux/9
  Demux4/3 -> Mux2/3
  Demux9/2 -> Mux1/8
  Demux9/3 -> Mux2/8
  Demux3/3 -> Mux2/2
  Demux9/1 -> Mux/8
  Demux10/2 -> Mux1/9
  Demux8/2 -> Mux1/7
  Demux3/1 -> Mux/2
  In6/1 -> Demux7/1
  Demux1/2 -> Mux1/1
  Demux6/1 -> Mux/5
  Demux8/1 -> Mux/7
  In1/1 -> Demux1/1
  In9/1 -> Demux10/1
  Demux7/1 -> Mux/6
  Demux1/1 -> Mux/1
  Demux3/2 -> Mux1/2
  Demux5/1 -> Mux/4
  Demux5/2 -> Mux1/4
  Demux6/2 -> Mux1/5
  Demux7/2 -> Mux1/6
  Mux/1 -> SOC/1  "SOC"
  In2/1 -> Demux3/1
  Mux2/1 -> voltage/1  "voltage"
  In3/1 -> Demux4/1
  In4/1 -> Demux5/1
  In8/1 -> Demux9/1

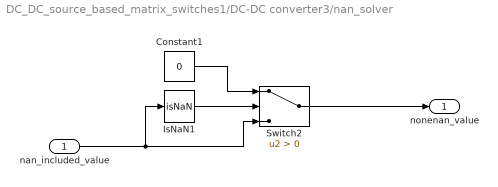
== system DC_DC_source_based_matrix_switches1/DC-DC converter3/nan_solver ==
  nan_included_value : Inport
  Constant1 : Constant  Value=0
  IsNaN1 : RelationalOperator  Operator=isNaN  OutDataTypeStr=boolean  RndMeth=Simplest  InputSameDT=off
  Switch2 : Switch  Criteria=u2 > Threshold  SaturateOnIntegerOverflow=off  InputSameDT=off
  nonenan_value : Outport
  wires:
  Constant1/1 -> Switch2/1
  nan_included_value/1 -> IsNaN1/1, Switch2/3
  IsNaN1/1 -> Switch2/2
  Switch2/1 -> nonenan_value/1

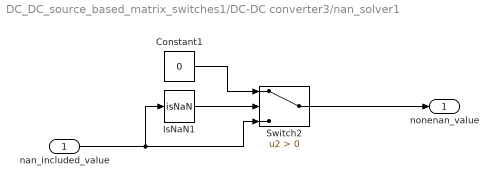
== system DC_DC_source_based_matrix_switches1/DC-DC converter3/nan_solver1 ==
  nan_included_value : Inport
  Constant1 : Constant  Value=0
  IsNaN1 : RelationalOperator  Operator=isNaN  OutDataTypeStr=boolean  RndMeth=Simplest  InputSameDT=off
  Switch2 : Switch  Criteria=u2 > Threshold  SaturateOnIntegerOverflow=off  InputSameDT=off
  nonenan_value : Outport
  wires:
  Switch2/1 -> nonenan_value/1
  IsNaN1/1 -> Switch2/2
  nan_included_value/1 -> Switch2/3, IsNaN1/1
  Constant1/1 -> Switch2/1

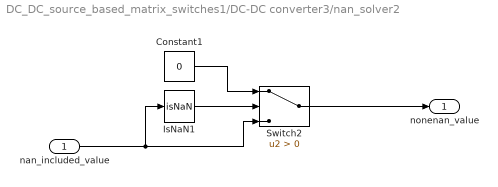
== system DC_DC_source_based_matrix_switches1/DC-DC converter3/nan_solver2 ==
  nan_included_value : Inport
  Constant1 : Constant  Value=0
  IsNaN1 : RelationalOperator  Operator=isNaN  OutDataTypeStr=boolean  RndMeth=Simplest  InputSameDT=off
  Switch2 : Switch  Criteria=u2 > Threshold  SaturateOnIntegerOverflow=off  InputSameDT=off
  nonenan_value : Outport
  wires:
  Constant1/1 -> Switch2/1
  nan_included_value/1 -> IsNaN1/1, Switch2/3
  IsNaN1/1 -> Switch2/2
  Switch2/1 -> nonenan_value/1

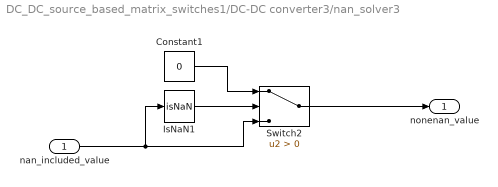
== system DC_DC_source_based_matrix_switches1/DC-DC converter3/nan_solver3 ==
  nan_included_value : Inport
  Constant1 : Constant  Value=0
  IsNaN1 : RelationalOperator  Operator=isNaN  OutDataTypeStr=boolean  RndMeth=Simplest  InputSameDT=off
  Switch2 : Switch  Criteria=u2 > Threshold  SaturateOnIntegerOverflow=off  InputSameDT=off
  nonenan_value : Outport
  wires:
  Switch2/1 -> nonenan_value/1
  IsNaN1/1 -> Switch2/2
  nan_included_value/1 -> Switch2/3, IsNaN1/1
  Constant1/1 -> Switch2/1

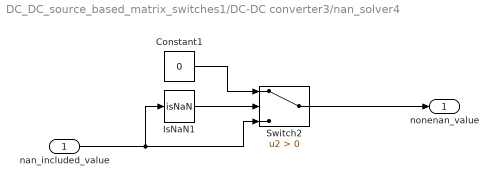
== system DC_DC_source_based_matrix_switches1/DC-DC converter3/nan_solver4 ==
  nan_included_value : Inport
  Constant1 : Constant  Value=0
  IsNaN1 : RelationalOperator  Operator=isNaN  OutDataTypeStr=boolean  RndMeth=Simplest  InputSameDT=off
  Switch2 : Switch  Criteria=u2 > Threshold  SaturateOnIntegerOverflow=off  InputSameDT=off
  nonenan_value : Outport
  wires:
  Constant1/1 -> Switch2/1
  nan_included_value/1 -> IsNaN1/1, Switch2/3
  IsNaN1/1 -> Switch2/2
  Switch2/1 -> nonenan_value/1

== system DC_DC_source_based_matrix_switches1/DC-DC converter3/nan_solver5 ==
  nan_included_value : Inport
  Constant1 : Constant  Value=0
  IsNaN1 : RelationalOperator  Operator=isNaN  OutDataTypeStr=boolean  RndMeth=Simplest  InputSameDT=off
  Switch2 : Switch  Criteria=u2 > Threshold  SaturateOnIntegerOverflow=off  InputSameDT=off
  nonenan_value : Outport
  wires:
  Switch2/1 -> nonenan_value/1
  IsNaN1/1 -> Switch2/2
  nan_included_value/1 -> Switch2/3, IsNaN1/1
  Constant1/1 -> Switch2/1

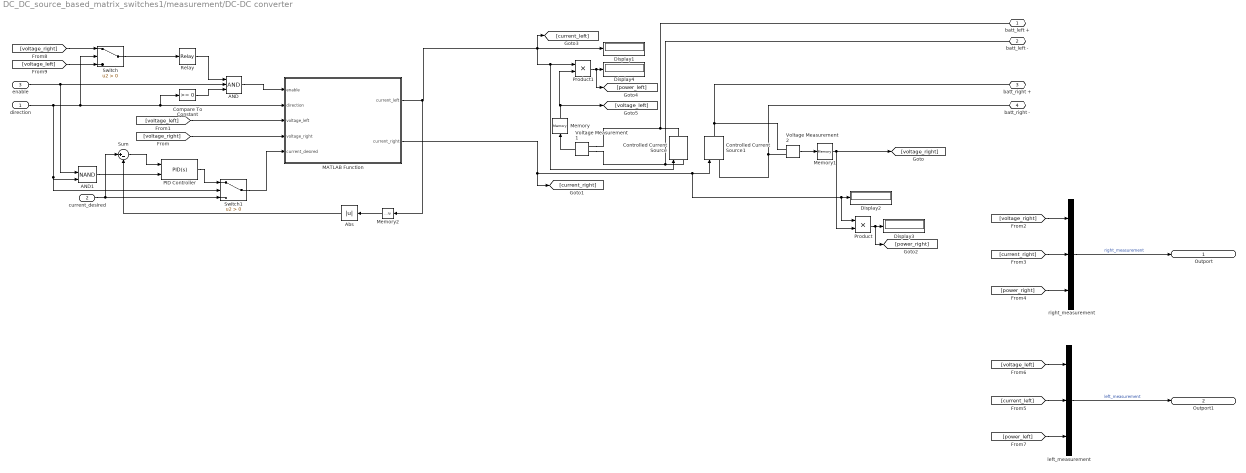
== system DC_DC_source_based_matrix_switches1/measurement/DC-DC converter ==
  direction : Inport
  current_desired : Inport  Port=2
  enable : Inport  Port=3
  AND : Logic  Inputs=3  IconShape=distinctive  AllPortsSameDT=off  OutDataTypeStr=boolean
  AND1 : Logic  Operator=NAND  IconShape=distinctive  AllPortsSameDT=off  OutDataTypeStr=boolean
  Abs : Abs  SaturateOnIntegerOverflow=off
  Compare To Constant : simulink/Logic and Bit Operations/Compare To Constant  relop=>=  const=0  OutDataTypeStr=boolean
  Controlled Current Source : spsControlledCurrentSourceLib/Controlled Current Source  Initialize=on  Source_Type=DC  Amplitude=0  Phase=0  Frequency=0  Measurements=None
  Controlled Current Source1 : spsControlledCurrentSourceLib/Controlled Current Source  Initialize=on  Source_Type=AC  Amplitude=0  Phase=0  Frequency=0  Measurements=None
  Display{1..4} (4 alike) : Display
  MATLAB Function : MATLAB Function  TreatAsAtomicUnit=on
  Memory : Memory
  Memory1 : Memory
  Memory2 : Memory
  PID Controller : slpidlib/PID Controller  Controller=PID  Form=Parallel  TimeDomain=Continuous-time  UseExternalTs=off  SampleTime=-1  IntegratorMethod=Forward Euler  FilterMethod=Forward Euler  ControllerParametersSource=internal  P=0.01  I=2  UseKiTs=off  D=0  N=100  UseFilter=on  TunerSelectOption=Transfer Function Based (PID Tuner App)  InitialConditionSource=internal  InitialConditionForIntegrator=0  InitialConditionForFilter=0  DifferentiatorICPrevScaledInput=0  ExternalReset=level  TrackingMode=off  Kt=1  LimitOutput=on  SatLimitsSource=internal  UpperSaturationLimit=2  LowerSaturationLimit=0  LinearizeAsGain=on  AntiWindupMode=none  Kb=1  LimitIntegrator=off  UpperIntegratorSaturationLimit=inf  LowerIntegratorSaturationLimit=-inf  POutMin=[]  POutMax=[]  IOutMin=[]  IOutMax=[]  DOutMin=[]  DOutMax=[]  NOutMin=[]  NOutMax=[]  SumOutMin=[]  SumOutMax=[]  SaturationOutMin=[]  SaturationOutMax=[]  PParamMin=[]  PParamMax=[]  IParamMin=[]  IParamMax=[]  DParamMin=[]  DParamMax=[]  NParamMin=[]  NParamMax=[]  KbParamMin=[]  KbParamMax=[]  KtParamMin=[]  KtParamMax=[]  KbOutMin=[]  KbOutMax=[]  KtOutMin=[]  KtOutMax=[]  IntegratorOutMin=[]  IntegratorOutMax=[]  FilterOutMin=[]  FilterOutMax=[]  SumI1OutMin=[]  SumI1OutMax=[]  SumI2OutMin=[]  SumI2OutMax=[]  SumI3OutMin=[]  SumI3OutMax=[]  SumI4OutMin=[]  SumI4OutMax=[]  SumDOutMin=[]  SumDOutMax=[]  DifferentiatorOutMin=[]  DifferentiatorOutMax=[]  FilterDiffOutCoefMin=[]  FilterDiffOutCoefMax=[]  ReciprocalOutMin=[]  ReciprocalOutMax=[]  SumDenOutMin=[]  SumDenOutMax=[]  SumNumOutMin=[]  SumNumOutMax=[]  DivideOutMin=[]  DivideOutMax=[]  UdiffTsProdOutMin=[]  UdiffTsProdOutMax=[]  NTsProdOutMin=[]  NTsProdOutMax=[]  UintegralTsProdOutMin=[]  UintegralTsProdOutMax=[]  UngainTsProdOutMin=[]  UngainTsProdOutMax=[]  ClampingZeroOutDataTypeStr=Inherit: Inherit via back propagation  ClampingZeroOutMin=[]  ClampingZeroOutMax=[]  FilterDenConstantOutDataTypeStr=Inherit: Inherit via back propagation  FilterDenConstantOutMin=[]  FilterDenConstantOutMax=[]  PCopyOutDataTypeStr=Inherit: Inherit via back propagation  PCopyOutMin=[]  PCopyOutMax=[]  NCopyOutDataTypeStr=Inherit: Inherit via back propagation  NCopyOutMin=[]  NCopyOutMax=[]  IntegratorContinuousStateAttributes=''  IntegratorStateMustResolveToSignalObject=off  IntegratorRTWStateStorageClass=Auto  FilterContinuousStateAttributes=''  FilterStateMustResolveToSignalObject=off  FilterRTWStateStorageClass=Auto  ParallelPVariant=InternalParameters  IdealPVariant=Disabled  IVariant=InternalParameters  DVariant=InternalParameters  IntegratorVariant=Continuous  SatVariant=Enabled  AWVariant=Passthrough  PCopyVariant=Disabled  TRVariant=Disabled  FdbkBlocksVariant=Forward  IdealPFdbkVariant=Disabled  SatFdbkVariant=Disabled  DerivativeFilterVariant=ContFilter  NVariant=InternalParameters  NCopyVariant=Disabled  FilterICVariant=InternalICsFilter  IntegratorICVariant=InternalICs  ExternalResetVariant=ExternalReset  TRSumVariant=Passthrough  SumFdbkVariant=Disabled  SumVariant=Sum_PID  TsampFilterVariant=InternalTs  TsampNgainVariant=Passthrough  TsampIntegralVariant=Disabled_SignalSpec  ExternalSaturationOutDataTypeStr=Inherit: Same as second input
  Product : Product
  Product1 : Product
  Relay : Relay  OnSwitchValue=3.5  OffSwitchValue=2
  Sum : Sum  Inputs=|+-
  Switch : Switch  Criteria=u2 > Threshold  SaturateOnIntegerOverflow=off  InputSameDT=off
  Switch1 : Switch  Criteria=u2 > Threshold  SaturateOnIntegerOverflow=off  InputSameDT=off
  Voltage Measurement1 : spsVoltageMeasurementLib/Voltage Measurement  PhasorSimulation=off  OutputType=Complex  PSBequivalent=0
  Voltage Measurement2 : spsVoltageMeasurementLib/Voltage Measurement  PhasorSimulation=off  OutputType=Complex  PSBequivalent=0
  left_measurement : Mux  Inputs=3
  right_measurement : Mux  Inputs=3
  batt_left + : PMIOPort  Side=Left
  batt_left - : PMIOPort  Port=2  Side=Left
  batt_right + : PMIOPort  Port=3  Side=Right
  batt_right - : PMIOPort  Port=4  Side=Right
  Outport : Outport
  Outport1 : Outport  Port=2
  wires:
  MATLAB Function/1(current_left) -> Memory2/1, Controlled Current Source/1, Product1/1, [current_left], Display1/1
  enable/1 -> AND1/1, AND/2
  Voltage Measurement2/1 -> Memory1/1
  direction/1 -> Compare To Constant/1, MATLAB Function/2(direction), Switch/2, AND1/2, Switch1/2
  [voltage_right] -> MATLAB Function/4(voltage_right)
  [voltage_left] -> MATLAB Function/3(voltage_left)
  Product/1 -> [power_right], Display3/1
  Product1/1 -> [power_left], Display4/1
  current_desired/1 -> Sum/1, Switch1/3
  [voltage_right] -> right_measurement/1
  [current_right] -> right_measurement/2
  [power_right] -> right_measurement/3
  [power_left] -> left_measurement/3
  [current_left] -> left_measurement/2
  [voltage_left] -> left_measurement/1
  right_measurement/1 -> Outport/1  "right_measurement"
  left_measurement/1 -> Outport1/1  "left_measurement"
  Voltage Measurement1/1 -> Memory/1
  Relay/1 -> AND/1
  AND/1 -> MATLAB Function/1(enable)
  Switch/1 -> Relay/1
  [voltage_left] -> Switch/3
  [voltage_right] -> Switch/1
  Memory/1 -> Product1/2, [voltage_left]
  Memory1/1 -> [voltage_right], Product/2
  Compare To Constant/1 -> AND/3
  Sum/1 -> PID Controller/1
  PID Controller/1 -> Switch1/1
  Switch1/1 -> MATLAB Function/5(current_desired)
  AND1/1 -> PID Controller/2
  Memory2/1 -> Abs/1
  MATLAB Function/2(current_right) -> [current_right], Product/1, Display2/1, Controlled Current Source1/1
  Abs/1 -> Sum/2
  connections:
  Voltage Measurement1/LConn1 -- batt_left +/RConn1 -- Controlled Current Source/RConn1
  Controlled Current Source1/RConn1 -- batt_right +/RConn1 -- Voltage Measurement2/LConn1
  Voltage Measurement2/LConn2 -- Controlled Current Source1/LConn1 -- batt_right -/RConn1
  Voltage Measurement1/LConn2 -- batt_left -/RConn1 -- Controlled Current Source/LConn1

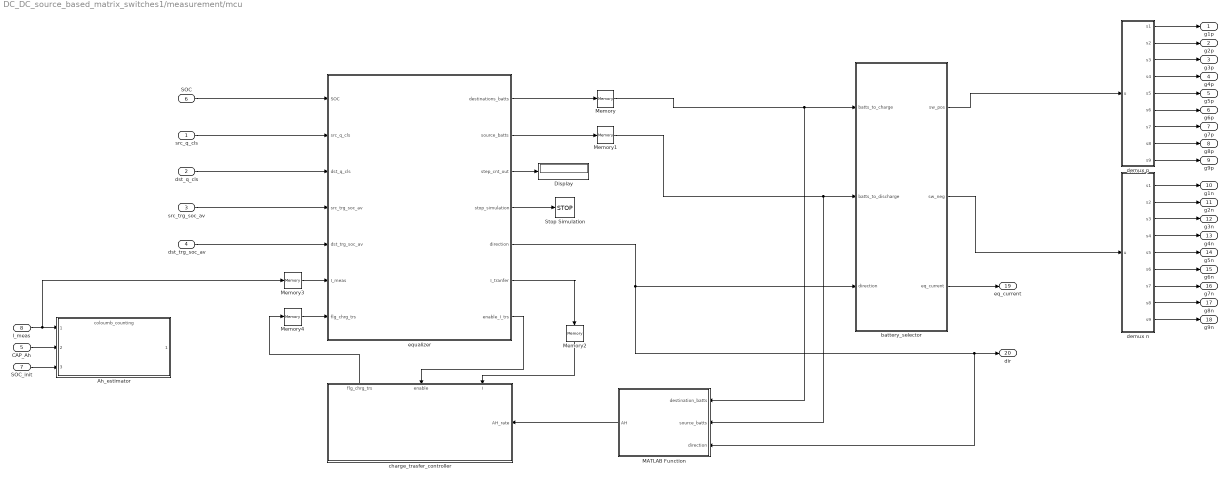
== system DC_DC_source_based_matrix_switches1/measurement/mcu ==
  src_q_cls : Inport
  dst_q_cls : Inport  Port=2
  src_trg_soc_av : Inport  Port=3
  dst_trg_soc_av : Inport  Port=4
  CAP_Ah : Inport  Port=5
  SOC : Inport  Port=6
  SOC_init : Inport  Port=7
  I_meas : Inport  Port=8
  Ah_estimator : ModelReference  ModelNameDialog=coloumb_counting.slx  SimulationMode=Normal  ModelReferenceVersion=2.1
  Display : Display
  MATLAB Function : MATLAB Function  TreatAsAtomicUnit=on
  Memory{,1..4} (5 alike) : Memory
  Stop Simulation : Stop
  battery_selector : MATLAB Function  TreatAsAtomicUnit=on
  charge_trasfer_controller : Subsystem
      settings: PortSchema="{\"entries\":[{\"content\":{\"sides\":[{\"content\":{},\"type\":\"ConnectorPlacement.EquallySpacedRectSide\",\"uuid\":\"48c70ec0-4261-4909-a719-c03e97c3e4ca\"},{\"content\":{\"connectorIds\":[\"In3\"],\"side\":\"RIGHT\"},\"type\":\"ConnectorPlacement.EquallySpacedRectSide\",\"uuid\":\"8a44a88a-c632-4005-90b8-1b0d09211c10\"},{\"content\":{\"connectorIds\":[\"Out1\",\"In1\",\"In2\"],\"side\":\"TOP\"},\"type\":\"ConnectorPlacement.EquallySpacedRectSide\",\"uuid\":\"71bafe47-820a-4a08-9919-e54bf550fba8\"}]},\"type\":\"ConnectorPlacement.EquallySpacedConnector\",\"uuid\":\"9c996bd2-099e-4131-a64b-67fbb4a72a45\"}],\"packageUris\":[\"http://schema.mathworks.com/mf0/Connector/R2020b\"],\"version\":\"1.0\"}"
  demux n : MATLAB Function  TreatAsAtomicUnit=on
  demux p : MATLAB Function  TreatAsAtomicUnit=on
  equalizer : MATLAB Function  TreatAsAtomicUnit=on
  g1p : Outport
  g2p : Outport  Port=2
  g3p : Outport  Port=3
  g4p : Outport  Port=4
  g5p : Outport  Port=5
  g6p : Outport  Port=6
  g7p : Outport  Port=7
  g8p : Outport  Port=8
  g9p : Outport  Port=9
  g1n : Outport  Port=10
  g2n : Outport  Port=11
  g3n : Outport  Port=12
  g4n : Outport  Port=13
  g5n : Outport  Port=14
  g6n : Outport  Port=15
  g7n : Outport  Port=16
  g8n : Outport  Port=17
  g9n : Outport  Port=18
  eq_current : Outport  Port=19
  dir : Outport  Port=20
  wires:
  battery_selector/3(eq_current) -> eq_current/1
  Memory/1 -> MATLAB Function/1(destination_batts), battery_selector/1(batts_to_charge)
  demux n/3(s3) -> g3n/1
  demux n/7(s7) -> g7n/1
  demux n/2(s2) -> g2n/1
  equalizer/1(destinations_batts) -> Memory/1
  dst_q_cls/1 -> equalizer/3(dst_q_cls)
  equalizer/4(stop_simulation) -> Stop Simulation/1
  demux p/7(s7) -> g7p/1
  Memory1/1 -> MATLAB Function/2(source_batts), battery_selector/2(batts_to_discharge)
  demux n/6(s6) -> g6n/1
  battery_selector/1(sw_pos) -> demux p/1(u)
  equalizer/2(source_batts) -> Memory1/1
  equalizer/3(step_cnt_out) -> Display/1
  battery_selector/2(sw_neg) -> demux n/1(u)
  src_q_cls/1 -> equalizer/2(src_q_cls)
  src_trg_soc_av/1 -> equalizer/4(src_trg_soc_av)
  demux n/5(s5) -> g5n/1
  demux n/8(s8) -> g8n/1
  dst_trg_soc_av/1 -> equalizer/5(dst_trg_soc_av)
  demux p/9(s9) -> g9p/1
  demux p/4(s4) -> g4p/1
  demux p/1(s1) -> g1p/1
  SOC/1 -> equalizer/1(SOC)
  demux p/5(s5) -> g5p/1
  demux p/2(s2) -> g2p/1
  demux p/8(s8) -> g8p/1
  demux n/1(s1) -> g1n/1
  demux n/4(s4) -> g4n/1
  demux n/9(s9) -> g9n/1
  demux p/3(s3) -> g3p/1
  demux p/6(s6) -> g6p/1
  SOC_init/1 -> Ah_estimator/3
  CAP_Ah/1 -> Ah_estimator/2
  MATLAB Function/1(AH) -> charge_trasfer_controller/3(AH_rate)
  equalizer/6(I_tranfer) -> Memory2/1
  equalizer/7(enable_I_trs) -> charge_trasfer_controller/1(enable)
  charge_trasfer_controller/1(flg_chrg_trs) -> Memory4/1
  equalizer/5(direction) -> MATLAB Function/3(direction), dir/1, battery_selector/3(direction)
  I_meas/1 -> Memory3/1, Ah_estimator/1
  Memory2/1 -> charge_trasfer_controller/2(I)
  Memory3/1 -> equalizer/6(I_meas)
  Memory4/1 -> equalizer/7(flg_chrg_trs)

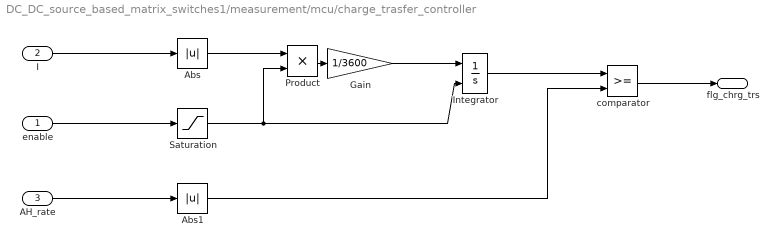
== system DC_DC_source_based_matrix_switches1/measurement/mcu/charge_trasfer_controller ==
  enable : Inport
  I : Inport  Port=2
  AH_rate : Inport  Port=3
  Abs : Abs  SaturateOnIntegerOverflow=off
  Abs1 : Abs  SaturateOnIntegerOverflow=off
  Gain : Gain  Gain=1/3600
  Integrator : Integrator  ExternalReset=either
  Product : Product
  Saturation : Saturate  UpperLimit=1  LowerLimit=0
  comparator : RelationalOperator  OutDataTypeStr=boolean  RndMeth=Simplest  InputSameDT=off
  flg_chrg_trs : Outport
  wires:
  comparator/1 -> flg_chrg_trs/1
  AH_rate/1 -> Abs1/1
  Abs/1 -> Product/1
  Integrator/1 -> comparator/1
  Product/1 -> Gain/1
  enable/1 -> Saturation/1
  Gain/1 -> Integrator/1
  Saturation/1 -> Product/2, Integrator/2
  I/1 -> Abs/1
  Abs1/1 -> comparator/2

== matlab function DC_DC_source_based_matrix_switches1/measurement/mcu/battery_selector ==
  data: batts_to_charge input; sw_pos output; sw_neg output; batts_to_discharge input; direction input; eq_current output
function [sw_pos, sw_neg, eq_current] = battery_selector(batts_to_charge, batts_to_discharge, direction)
    sw_pos = 0;
    sw_neg = 0;
    eq_current = 0;
    eq_current_tmp = 0;
% to prevent invalid switch selection
if ( batts_to_charge(1, 1) <= batts_to_charge(1, 2) && ...
     batts_to_discharge(1, 1) <= batts_to_discharge(1, 2))
    
    % charge the capacitor using batteries
    if(direction == 0)
        sw_pos = batts_to_discharge(1, 1);
        sw_neg = batts_to_discharge(1, 2);
        eq_current_tmp = 2;        
    % charge the battery using capacitor
    elseif(direction == 1)
        sw_pos = batts_to_charge(1, 1);
        sw_neg = batts_to_charge(1, 2);
        eq_current_tmp = 2;
    else
        sw_pos = 0;
        sw_neg = 0;

    end


    eq_current = eq_current_tmp * 0.5;

end


end

== matlab function DC_DC_source_based_matrix_switches1/measurement/mcu/demux n ==
  data: u input; s1 output; s2 output; s3 output; s4 output; s5 output; s6 output; s7 output; s8 output; s9 output
function [s1, s2, s3, s4, s5, s6, s7, s8, s9] = demux(u)

    switch(u)
        case 1
            s1 = 1; s2 = 0;	s3 = 0; s4 = 0; s5 = 0; s6 = 0; s7 = 0; s8 = 0; s9 = 0;
        case 2      	
            s1 = 0; s2 = 1;	s3 = 0; s4 = 0; s5 = 0; s6 = 0; s7 = 0; s8 = 0; s9 = 0;
        case 3      	
            s1 = 0; s2 = 0;	s3 = 1; s4 = 0; s5 = 0; s6 = 0; s7 = 0; s8 = 0; s9 = 0;
        case 4      	
            s1 = 0; s2 = 0;	s3 = 0; s4 = 1; s5 = 0; s6 = 0; s7 = 0; s8 = 0; s9 = 0;
        case 5      	
            s1 = 0; s2 = 0;	s3 = 0; s4 = 0; s5 = 1; s6 = 0; s7 = 0; s8 = 0; s9 = 0;
        case 6      	
            s1 = 0; s2 = 0;	s3 = 0; s4 = 0; s5 = 0; s6 = 1; s7 = 0; s8 = 0; s9 = 0;
        case 7      
            s1 = 0; s2 = 0;	s3 = 0; s4 = 0; s5 = 0; s6 = 0; s7 = 1; s8 = 0; s9 = 0;
        case 8      	
            s1 = 0; s2 = 0;	s3 = 0; s4 = 0; s5 = 0; s6 = 0; s7 = 0; s8 = 1; s9 = 0;
        case 9      
            s1 = 0; s2 = 0;	s3 = 0; s4 = 0; s5 = 0; s6 = 0; s7 = 0; s8 = 0; s9 = 1;
        otherwise   	
            s1 = 0; s2 = 0;	s3 = 0; s4 = 0; s5 = 0; s6 = 0; s7 = 0; s8 = 0; s9 = 0;
    end
end

== matlab function DC_DC_source_based_matrix_switches1/measurement/mcu/demux p ==
  data: u input; s1 output; s2 output; s3 output; s4 output; s5 output; s6 output; s7 output; s8 output; s9 output
function [s1, s2, s3, s4, s5, s6, s7, s8, s9] = demux(u)

    switch(u)
        case 1
            s1 = 1; s2 = 0;	s3 = 0; s4 = 0; s5 = 0; s6 = 0; s7 = 0; s8 = 0; s9 = 0;
        case 2      	
            s1 = 0; s2 = 1;	s3 = 0; s4 = 0; s5 = 0; s6 = 0; s7 = 0; s8 = 0; s9 = 0;
        case 3      	
            s1 = 0; s2 = 0;	s3 = 1; s4 = 0; s5 = 0; s6 = 0; s7 = 0; s8 = 0; s9 = 0;
        case 4      	
            s1 = 0; s2 = 0;	s3 = 0; s4 = 1; s5 = 0; s6 = 0; s7 = 0; s8 = 0; s9 = 0;
        case 5      	
            s1 = 0; s2 = 0;	s3 = 0; s4 = 0; s5 = 1; s6 = 0; s7 = 0; s8 = 0; s9 = 0;
        case 6      	
            s1 = 0; s2 = 0;	s3 = 0; s4 = 0; s5 = 0; s6 = 1; s7 = 0; s8 = 0; s9 = 0;
        case 7      
            s1 = 0; s2 = 0;	s3 = 0; s4 = 0; s5 = 0; s6 = 0; s7 = 1; s8 = 0; s9 = 0;
        case 8      	
            s1 = 0; s2 = 0;	s3 = 0; s4 = 0; s5 = 0; s6 = 0; s7 = 0; s8 = 1; s9 = 0;
        case 9      
            s1 = 0; s2 = 0;	s3 = 0; s4 = 0; s5 = 0; s6 = 0; s7 = 0; s8 = 0; s9 = 1;
        otherwise   	
            s1 = 0; s2 = 0;	s3 = 0; s4 = 0; s5 = 0; s6 = 0; s7 = 0; s8 = 0; s9 = 0;
    end
end

== matlab function DC_DC_source_based_matrix_switches1/measurement/mcu/equalizer ==
  data: destinations_batts output; SOC input; source_batts output [..50]; src_q_cls input; dst_q_cls input; src_trg_soc_av input; dst_trg_soc_av input; I_meas input; step_cnt_out output; stop_simulation output; direction output; I_tranfer output; enable_I_trs output; flg_chrg_trs input
function [destinations_batts, source_batts, step_cnt_out, stop_simulation, direction, I_tranfer, enable_I_trs] = battery_selector(SOC, src_q_cls, dst_q_cls, src_trg_soc_av, dst_trg_soc_av, I_meas, flg_chrg_trs)


I_tranfer  = 0;
stop_simulation  = 0;
source_batts = [0 0];
destinations_batts = [0 0];
dst_trg_soc_av_tmp = dst_trg_soc_av;
src_trg_soc_av_tmp = src_trg_soc_av;

dst_trg_soc_av_tmp(dst_trg_soc_av == 0) = Inf;
% src_trg_soc_av_tmp(src_trg_soc_av == 0) = Inf;
% the number of steps to equlalize the battery pack
step = length(src_q_cls);

persistent step_cnt;
persistent I_cells_source;
persistent I_cells_destination;
persistent dir;
persistent enable;



if isempty(step_cnt)
    step_cnt = 1;
    assert(1, 'Simulation terminated because x >= 10')

end

if isempty(I_cells_source)
    I_cells_source = 0;
end
if isempty(I_cells_destination)
    I_cells_destination = 0;
end
if isempty(dir)
    dir = -1;
end
if isempty(enable)
    enable = 0;
end



soc = SOC';
if src_q_cls(step_cnt, :) > 0


    source_batts = src_q_cls(step_cnt, :);
    I_cells_source = I_meas(source_batts(1, 1));       % source cells current
    destinations_batts = dst_q_cls(step_cnt, :);
    I_cells_destination = I_meas(destinations_batts(1, 1));  % destication cells current



    if(dir == -1 && flg_chrg_trs == 0) % dischaege source if in the begining of charge transfering
        I_tranfer = I_cells_source;
        enable = 1; % start counting coulombs
        dir = 0; 
    end
    if(dir == 0)
        I_tranfer = I_cells_source;
    end

    if(dir == 0 && flg_chrg_trs == 1 && enable == 1) % reset the flag
        enable = 0;
    end

    if(dir == 0 && flg_chrg_trs == 0 && enable == 0) % charge the destination if the prevoius charge transfer terminated
        I_tranfer = I_cells_destination;
        enable = 1;
        dir = 1;
    end
    if(dir == 1)
        I_tranfer = I_cells_destination;
    end

    if(dir == 1 && flg_chrg_trs == 1 && enable == 1) % reset the flag
        enable = 0;
    end

    if(dir == 1 && flg_chrg_trs == 0 && enable == 0) % charge transfer terminated
        dir = -1;
    end
    
    sm = mean(soc(src_q_cls(step_cnt, 1):src_q_cls(step_cnt, 2)));
    dm = mean(soc(dst_q_cls(step_cnt, 1):dst_q_cls(step_cnt, 2)));
    if(sm <= src_trg_soc_av_tmp(step_cnt) || dm >= dst_trg_soc_av_tmp(step_cnt)) && dir == -1
        step_cnt = step_cnt + 1;
    end
else
    direction = 0;
    I_cells_source = 0;
    I_cells_destination = 0;
    dir = -1;
    stop_simulation  = 1;
    enable = 0
end
direction = dir;
enable_I_trs = enable;


step_cnt_out = step_cnt;

end

== matlab function DC_DC_source_based_matrix_switches1/mcu/queue_handler ==
  data: src_q_cls input; source_batts output; dst_q_cls input; src_trg_soc_av input; dst_trg_soc_av input; destinations_batts output; src_trg_soc_av_o output size=1; dst_trg_soc_av_o output size=1; SOC input; stop_transfer input; stop_simulation output
function [source_batts ,destinations_batts, src_trg_soc_av_o, dst_trg_soc_av_o, stop_simulation] = fcn(src_q_cls, dst_q_cls, src_trg_soc_av, dst_trg_soc_av, SOC, stop_transfer)

I_tranfer  = 0;
stop_simulation = 0;
source_batts = [0 0];
destinations_batts = [0 0];
dst_trg_soc_av_tmp = dst_trg_soc_av;
src_trg_soc_av_tmp = src_trg_soc_av;
soc = zeros(1, 9);

src_trg_soc_av_o = 0;
dst_trg_soc_av_o = 0;



dst_trg_soc_av_tmp(dst_trg_soc_av == 0) = 255;
%src_trg_soc_av_tmp(src_trg_soc_av == 0) = 255;

% the number of steps to equlalize the battery pack
step = length(src_q_cls);

persistent step_cnt;
persistent I_cells_source;
persistent I_cells_destination;

if isempty(step_cnt)
    step_cnt = 1;
    assert(1, 'Simulation terminated because x >= 10')
end

if isempty(I_cells_source)
    I_cells_source = 0;
end
if isempty(I_cells_destination)
    I_cells_destination = 0;
end


src_trg_soc_av_o = src_trg_soc_av_tmp(step_cnt); 
dst_trg_soc_av_o = dst_trg_soc_av_tmp(step_cnt); 




soc = SOC';
if src_q_cls(step_cnt, :) > 0


    source_batts = src_q_cls(step_cnt, :);
    %I_cells_source = I_meas(source_batts(1, 1));       % source cells current
    destinations_batts = dst_q_cls(step_cnt, :);
    %I_cells_destination = I_meas(destinations_batts(1, 1));  % destication cells current

    
    %sm = mean(soc(src_q_cls(step_cnt, 1):src_q_cls(step_cnt, 2)));
    %dm = mean(soc(dst_q_cls(step_cnt, 1):dst_q_cls(step_cnt, 2)));
    %if(sm <= src_trg_soc_av_tmp(step_cnt) || dm >= dst_trg_soc_av_tmp(step_cnt))
   
    if stop_transfer
        step_cnt = step_cnt + 1;   
    end

else
    stop_simulation = 1;
end
